simulink model "standard"  (R2017b)
settings: Solver=FixedStepDiscrete  StartTime=0.0  StopTime=inf  RelTol=1e-3  EnableMultiTasking=on
model workspace (MAT data in the model file):
  cfg_native : struct (value not decoded)
  en_add_channels = 127
  host_ip = 2130706433
  host_port = 50223
  local_ip = 2130706433
  local_port = 50224
  num_en_channels = 8
  num_samples = 8
  sample_rate = 500
  serial_number = 'NB-2016.09.83'
undefined symbols (not defined in the file): NB
libraries: gtecHighspeedLib x9, dspnetwork x3, gNautilusLib x1, gNautilusTools x1
settings Model: Creator=g.tec Maresch  LastModifiedBy=Gabriel
settings DataIOCC: LimitDataPoints=on  SaveFormat=Array
settings OptimizationCC: ExpressionDepthLimit=2147483647  LifeSpan=inf
settings DebuggingCC: UnderspecifiedInitializationDetection=Classic  MergeDetectMultiDrivingBlocksExec=none  SolverPrmCheckMsg=warning  FcnCallInpInsideContextMsg=warning  FrameProcessingCompatibilityMsg=none  StateNameClashWarn=warning  SFUnexpectedBacktrackingDiag=warning  SFNoUnconditionalDefaultTransitionDiag=warning  SFExecutionAtInitializationDiag=none
settings HardwareCC: ProdBitPerInt=16  ProdBitPerPointer=16  ProdBitPerSizeT=16  ProdBitPerPtrDiffT=16  ProdLargestAtomicFloat=None  ProdEndianess=Unspecified  ProdWordSize=8  ProdShiftRightIntArith=off  ProdHWDeviceType=Intel->8051 Compatible
settings ModelReferenceCC: PropagateSignalLabelsOutOfModel=off
settings SFSimCC: SFSimEcho=off  SimCtrlC=off  SimIntegrity=off
settings CodeAppCC: StateflowObjectComments=on
settings GRTTargetCC: TargetLangStandard=C89/C90 (ANSI)  GeneratePreprocessorConditionals=Disable all  CombineOutputUpdateFcns=off  GRTInterface=on
settings ConfigComp: CovMetricSettings=dw  CovHtmlReporting=on  CovSaveCumulativeToWorkspaceVar=on  CovSaveSingleToWorkspaceVar=on  CovExternalEMLEnable=off

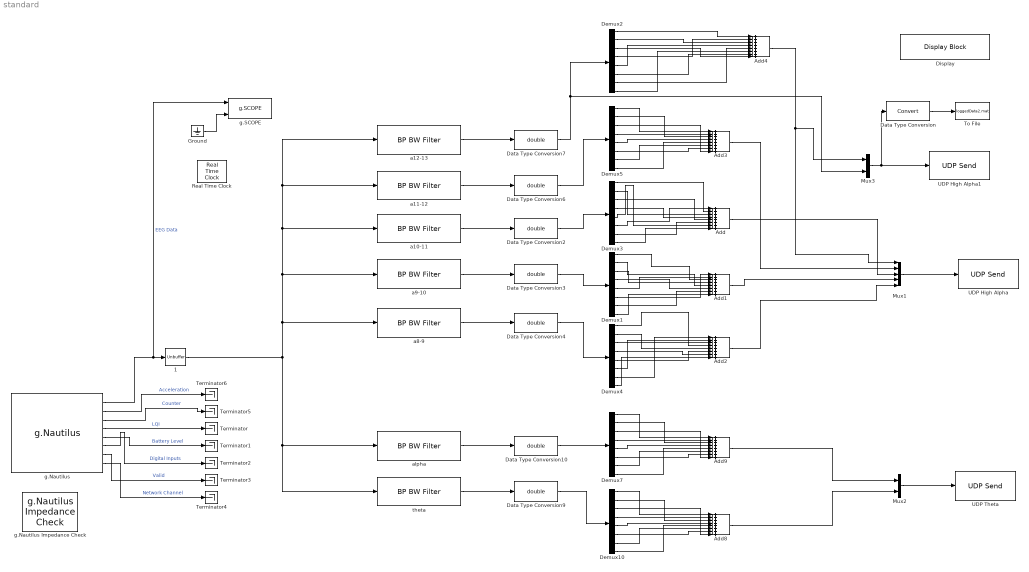
== system standard ==
  1 : Unbuffer
  Add{,1..4,8..9} (7 alike) : Sum  Inputs=++++++++
  Data Type Conversion : DataTypeConversion
  Data Type Conversion{2..4,6..7,9..10} (7 alike) : DataTypeConversion  OutDataTypeStr=double
  Demux{1..5,7,10} (7 alike) : Demux  Outputs=8
  Display : DisplayBlock  WebBlockId=140  ModelName=standard  LabelPosition=Hide  ShowInitialText=on  ShowFormattedStrings=off  Format=long  Alignment=Center
  Ground : Ground
  Mux1 : Mux  Inputs=5
  Mux2 : Mux  Inputs=2
  Mux3 : Mux  Inputs=2
  Real Time Clock : gtecHighspeedLib/Real Time Clock  timeprofile=on
      settings: SourceProductName=g.tec Highspeed Library
  Terminator{,1..6} (7 alike) : Terminator
  To File : ToFile  Filename=loggedData2.mat  MatrixName=z
  UDP High Alpha : dspnetwork/UDP Send  remoteURL='192.168.0.2'  remotePort=25000  localURL='0.0.0.0'  localPortSource=Automatically determine  localPort=-1  sampletime=-1  blockPlatform=[]  separateLengthPort=0
      settings: SourceProductName=DSP System Toolbox  SourceProductBaseCode=DS
  UDP High Alpha1 : dspnetwork/UDP Send  remoteURL='192.168.0.2'  remotePort=27000  localURL='0.0.0.0'  localPortSource=Automatically determine  localPort=-1  sampletime=-1  blockPlatform=[]  separateLengthPort=0
      settings: SourceProductName=DSP System Toolbox  SourceProductBaseCode=DS
  UDP Theta : dspnetwork/UDP Send  remoteURL='192.168.0.2'  remotePort=26000  localURL='0.0.0.0'  localPortSource=Automatically determine  localPort=-1  sampletime=-1  blockPlatform=[]  separateLengthPort=0
      settings: SourceProductName=DSP System Toolbox  SourceProductBaseCode=DS
  "a10-11  " : gtecHighspeedLib/BP BW Filter    LPOrder=3  UpperFreq=13  HPOrder=3  LowerFreq=12  SampFreq=250
      settings: SourceProductName=g.tec Highspeed Library
  a11-12 : gtecHighspeedLib/BP BW Filter    LPOrder=3  UpperFreq=13  HPOrder=3  LowerFreq=12  SampFreq=250
      settings: SourceProductName=g.tec Highspeed Library
  a12-13 : gtecHighspeedLib/BP BW Filter    LPOrder=3  UpperFreq=13  HPOrder=3  LowerFreq=12  SampFreq=250
      settings: SourceProductName=g.tec Highspeed Library
  a8-9 : gtecHighspeedLib/BP BW Filter    LPOrder=3  UpperFreq=9  HPOrder=3  LowerFreq=8  SampFreq=250
      settings: SourceProductName=g.tec Highspeed Library
  "a9-10 " : gtecHighspeedLib/BP BW Filter    LPOrder=3  UpperFreq=32  HPOrder=3  LowerFreq=13  SampFreq=250
      settings: SourceProductName=g.tec Highspeed Library
  alpha : gtecHighspeedLib/BP BW Filter    LPOrder=3  UpperFreq=13  HPOrder=3  LowerFreq=8  SampFreq=250
      settings: SourceProductName=g.tec Highspeed Library
  g.Nautilus : gNautilusLib/g.Nautilus  Tag=g.Nautilus  Description=Operates a g.Nautilus device and provides acquired data on its outputs.  sample_rate=500  local_ip=2130706433  local_port=50224  host_ip=2130706433  host_port=50223  serial_number=NB-2016.09.83  num_samples=8  num_en_channels=8  add_channels=127
      settings: SourceProductName=g.Nautilus
  g.Nautilus Impedance Check : gNautilusTools/g.Nautilus Impedance Check
  g.SCOPE : gtecHighspeedLib/g.SCOPE
      settings: SourceProductName=g.tec Highspeed Library
  theta : gtecHighspeedLib/BP BW Filter    LPOrder=3  UpperFreq=8  HPOrder=3  LowerFreq=4  SampFreq=250
      settings: SourceProductName=g.tec Highspeed Library
  wires:
  g.Nautilus/1 -> g.SCOPE/1, 1/1  "EEG Data"
  g.Nautilus/8 -> Terminator4/1  "Network Channel"
  g.Nautilus/7 -> Terminator3/1  "Valid"
  g.Nautilus/6 -> Terminator2/1  "Digital Inputs"
  g.Nautilus/5 -> Terminator1/1  "Battery Level"
  g.Nautilus/4 -> Terminator/1  "LQI"
  g.Nautilus/3 -> Terminator5/1  "Counter"
  g.Nautilus/2 -> Terminator6/1  "Acceleration"
  "a10-11  "/1 -> Data Type Conversion2/1
  "a9-10 "/1 -> Data Type Conversion3/1
  a8-9/1 -> Data Type Conversion4/1
  Data Type Conversion2/1 -> Demux3/1
  Demux3/1 -> Add/2
  Demux3/2 -> Add/3
  Demux3/3 -> Add/5
  Demux3/4 -> Add/4
  Demux3/5 -> Add/7
  Demux3/6 -> Add/1
  Data Type Conversion3/1 -> Demux1/1
  Demux1/1 -> Add1/3
  Demux1/2 -> Add1/5
  Demux1/3 -> Add1/4
  Demux1/4 -> Add1/6
  Demux1/5 -> Add1/2
  Demux1/6 -> Add1/1
  Demux4/1 -> Add2/4
  Demux4/2 -> Add2/5
  Demux4/3 -> Add2/3
  Demux4/4 -> Add2/7
  Demux4/5 -> Add2/6
  Demux4/6 -> Add2/2
  Data Type Conversion4/1 -> Demux4/1
  Demux3/7 -> Add/6
  Demux3/8 -> Add/8
  Demux4/8 -> Add2/8
  Demux4/7 -> Add2/1
  Demux1/7 -> Add1/7
  Demux1/8 -> Add1/8
  Add/1 -> Mux1/3
  Add1/1 -> Mux1/4
  Add2/1 -> Mux1/5
  Ground/1 -> g.SCOPE/2
  Mux1/1 -> UDP High Alpha/1
  a12-13/1 -> Data Type Conversion7/1
  a11-12/1 -> Data Type Conversion6/1
  Data Type Conversion6/1 -> Demux5/1
  Demux5/8 -> Add3/5
  Demux5/7 -> Add3/6
  Demux5/6 -> Add3/7
  Demux5/5 -> Add3/4
  Demux5/4 -> Add3/2
  Demux5/2 -> Add3/3
  Demux5/1 -> Add3/1
  Demux5/3 -> Add3/8
  Demux2/3 -> Add4/8
  Demux2/4 -> Add4/2
  Demux2/6 -> Add4/7
  Demux2/5 -> Add4/4
  Data Type Conversion7/1 -> Mux3/2, Demux2/1
  Demux2/1 -> Add4/1
  Demux2/2 -> Add4/3
  Add3/1 -> Mux1/2
  Demux7/7 -> Add9/6
  Mux2/1 -> UDP Theta/1
  Demux10/6 -> Add8/7
  Demux10/4 -> Add8/2
  Demux10/7 -> Add8/6
  Data Type Conversion9/1 -> Demux10/1
  Demux10/8 -> Add8/5
  Data Type Conversion10/1 -> Demux7/1
  Demux10/5 -> Add8/4
  1/1 -> theta/1, alpha/1, a8-9/1, "a9-10 "/1, a12-13/1, a11-12/1, "a10-11  "/1
  Demux7/1 -> Add9/1
  Demux7/5 -> Add9/4
  theta/1 -> Data Type Conversion9/1
  Demux7/4 -> Add9/2
  Demux7/6 -> Add9/7
  Demux7/3 -> Add9/8
  Demux10/3 -> Add8/8
  alpha/1 -> Data Type Conversion10/1
  Demux7/8 -> Add9/5
  Add8/1 -> Mux2/2
  Demux10/2 -> Add8/3
  Demux7/2 -> Add9/3
  Add9/1 -> Mux2/1
  Demux10/1 -> Add8/1
  Add4/1 -> Mux3/1, Mux1/1
  Demux2/7 -> Add4/5
  Demux2/8 -> Add4/6
  Mux3/1 -> Data Type Conversion/1, UDP High Alpha1/1
  Data Type Conversion/1 -> To File/1
